simulink model "Lab3_Buck_Chopper"  (R2016b)
settings: Solver=VariableStepAuto  StartTime=0.0  StopTime=10.0  RelTol=1e-3  EnableMultiTasking=on
libraries: powerlib x7
settings Model: Creator=Yash Bansod  LastModifiedBy=Yash Bansod
settings DataIOCC: LimitDataPoints=on
settings OptimizationCC: LifeSpan=inf
settings DebuggingCC: AllowSymbolicDim=off  SFUnexpectedBacktrackingDiag=warning  SFNoUnconditionalDefaultTransitionDiag=warning  SFExecutionAtInitializationDiag=none
settings ModelReferenceCC: PropagateSignalLabelsOutOfModel=off
settings GRTTargetCC: TargetLangStandard=C89/C90 (ANSI)
settings ConfigComp: CovMetricSettings=dw  CovHtmlReporting=on  CovSaveCumulativeToWorkspaceVar=on  CovSaveSingleToWorkspaceVar=on  CovExternalEMLEnable=off

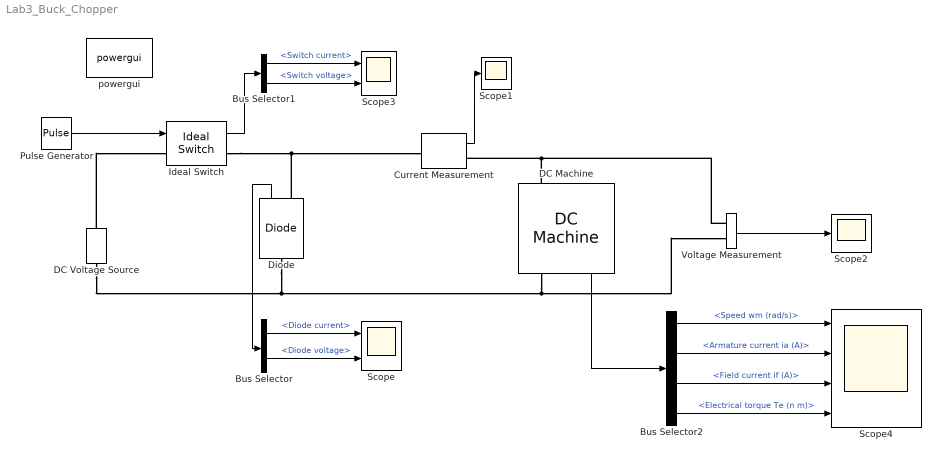
== system Lab3_Buck_Chopper ==
  Bus Selector : BusSelector  OutputSignals=Diode current,Diode voltage
  Bus Selector1 : BusSelector  OutputSignals=Switch current,Switch voltage
  Bus Selector2 : BusSelector  OutputSignals=Speed wm (rad/s),Armature current ia (A),Field current if (A),Electrical torque Te (n m)
  Current Measurement : powerlib/Measurements/Current Measurement  PhasorSimulation=off  OutputType=Complex  PSBequivalent=0
  DC Machine : powerlib/Machines/DC Machine  PresetModel=No  MechanicalLoad=Torque TL  FieldType=Permanent magnet  ShowDetailedParameters=on  MeasurementBus=off  RLa="[ 1  0.5]"  RLf="[ 240  120]"  Laf=1.8  MachineConstant=Torque constant (N.m/A)  Ke=0.0954  Kt=0.01  J=0.01  Bm=0.1  Tf=0  w0=0  Ifinit=0  TsPowergui=0  TsBlock=-1
  DC Voltage Source : powerlib/Electrical Sources/DC Voltage Source  Amplitude=220  Measurements=Voltage
  Diode : powerlib/Power Electronics/Diode  Ron=0.001  Lon=0  Vf=0.8  IC=0  UseSnubber=off  Rs=500  Cs=250e-9  Measurements=on
  Ideal Switch : powerlib/Power Electronics/Ideal Switch  Ron=0.001  Lon=0  IC=0  Rs=1e5  Cs=inf  Measurements=on
  Pulse Generator : DiscretePulseGenerator  PulseType=Time based  Period=0.001  PulseWidth=50
  Scope : Scope  NumInputPorts=2
  Scope1 : Scope
  Scope2 : Scope
  Scope3 : Scope  NumInputPorts=2
  Scope4 : Scope  NumInputPorts=4
  Voltage Measurement : powerlib/Measurements/Voltage Measurement  PhasorSimulation=off  OutputType=Complex  PSBequivalent=0
  powergui : powerlib/powergui  Priority=1  SimulationMode=Continuous  SolverType=Tustin/Backward Euler (TBE)  SampleTime=50e-6  frequency=60  SPID=on  DisableSnubberDevices=off  DisableRonSwitches=off  DisableVfSwitches=off  SwTol=0  DisplayEquations=off  Interpol=off  ExternalGateDelay=off  methode=off  Ts=10  FunctionMessages=off  echomessages=off  HookPort=off  EnableUseOfTLC=off  x0status=blocks  frequencyindice=0  Pbase=100e6  ErrMax=1e-4  Iterations=50  UnitsV=kV  UnitsW=MW  buscounter=0  RestoreLinks=warning  ResistiveCurrentMeasurement=off  Frange=[0:2:500]  Ylog=off  Xlog=on  ShowGrid=off  save=off  variable=ZData  structure=0  ZoomFFT=off  StartTime=0.0  cycles=1  DisplayStyle=1  fundamental=60  FreqAxis=off  MaxFrequency=1000  frequencyindicesteady=1  RmsSteady=1  display=off
  wires:
  Pulse Generator/1 -> Ideal Switch/1
  Diode/1 -> Bus Selector/1
  Bus Selector/1 -> Scope/1  "<Diode current>"
  Bus Selector/2 -> Scope/2  "<Diode voltage>"
  Current Measurement/1 -> Scope1/1
  Voltage Measurement/1 -> Scope2/1
  Ideal Switch/1 -> Bus Selector1/1
  Bus Selector1/1 -> Scope3/1  "<Switch current>"
  Bus Selector1/2 -> Scope3/2  "<Switch voltage>"
  DC Machine/1 -> Bus Selector2/1
  Bus Selector2/1 -> Scope4/1  "<Speed wm (rad/s)>"
  Bus Selector2/2 -> Scope4/2  "<Armature current ia (A)>"
  Bus Selector2/3 -> Scope4/3  "<Field current if (A)>"
  Bus Selector2/4 -> Scope4/4  "<Electrical torque Te (n m)>"
  connections:
  DC Machine/LConn1 -- Voltage Measurement/LConn1 -- Current Measurement/RConn1
  DC Voltage Source/LConn1 -- Diode/LConn1 -- Voltage Measurement/LConn2 -- DC Machine/RConn1
  DC Voltage Source/RConn1 -- Ideal Switch/LConn1
  Ideal Switch/RConn1 -- Current Measurement/LConn1 -- Diode/RConn1
